simulink model "merohid"  (Simulink 7.6)
settings: Solver=ode45  StartTime=0.0  StopTime=10.0  RelTol=1e-3
libraries: fl_lib x6, elec_lib x1, nesl_utility x1
settings Model: Creator=Fodi  LastModifiedBy=Fodi

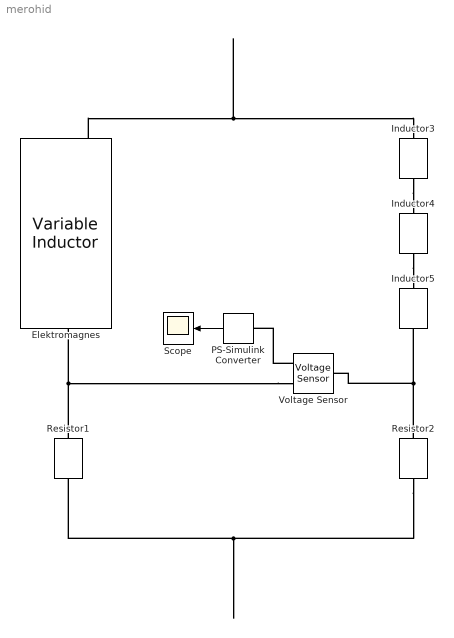
== system merohid ==
  Elektromagnes : elec_lib/Passive Devices/Variable Inductor  DialogController=NetworkEngine.DynNeDlgSource  SystemSampleTime=-1  prm=1  Lmin=1e-6 H  g=1e-9 1/Ohm  i0=0 A  phi0=0 Wb  LocalVarLogging=[]
  Inductor3 : fl_lib/Electrical/Electrical Elements/Inductor  DialogController=NetworkEngine.DynNeDlgSource  SystemSampleTime=-1  l=1e-6 H  i0=0 A  r=0 Ohm  g=1e-9 1/Ohm  i_Log=off  v_Log=off  i_L_Log=off  LocalVarNames=|i|v|i_L  LocalVarDescs=|i|v|Internal variable for current through inductor term  LocalVarLogging=[0 0 0]
  Inductor4 : fl_lib/Electrical/Electrical Elements/Inductor  DialogController=NetworkEngine.DynNeDlgSource  SystemSampleTime=-1  l=1e-6 H  i0=0 A  r=0 Ohm  g=1e-9 1/Ohm  i_Log=off  v_Log=off  i_L_Log=off  LocalVarNames=|i|v|i_L  LocalVarDescs=|i|v|Internal variable for current through inductor term  LocalVarLogging=[0 0 0]
  Inductor5 : fl_lib/Electrical/Electrical Elements/Inductor  DialogController=NetworkEngine.DynNeDlgSource  SystemSampleTime=-1  l=1e-6 H  i0=0 A  r=0 Ohm  g=1e-9 1/Ohm  i_Log=off  v_Log=off  i_L_Log=off  LocalVarNames=|i|v|i_L  LocalVarDescs=|i|v|Internal variable for current through inductor term  LocalVarLogging=[0 0 0]
  PS-Simulink Converter : nesl_utility/PS-Simulink Converter  DialogController=NetworkEngine.DynNeUtilDlgSource  SystemSampleTime=-1  PhysicalDomain=network_engine_domain  LeftPortType=input  RightPortType=output  SubClassName=ps_output  Unit=1  AffineConversion=off
  Resistor1 : fl_lib/Electrical/Electrical Elements/Resistor  DialogController=NetworkEngine.DynNeDlgSource  SystemSampleTime=-1  R=1 Ohm  i_Log=off  v_Log=off  LocalVarNames=|i|v  LocalVarDescs=|i|v  LocalVarLogging=[0 0]
  Resistor2 : fl_lib/Electrical/Electrical Elements/Resistor  DialogController=NetworkEngine.DynNeDlgSource  SystemSampleTime=-1  R=1 Ohm  i_Log=off  v_Log=off  LocalVarNames=|i|v  LocalVarDescs=|i|v  LocalVarLogging=[0 0]
  Scope : Scope
  Voltage Sensor : fl_lib/Electrical/Electrical Sensors/Voltage Sensor  DialogController=NetworkEngine.DynNeDlgSource  SystemSampleTime=-1  i1_Log=off  v1_Log=off  LocalVarNames=|i1|v1  LocalVarDescs=|i1|v1  LocalVarLogging=[0 0]
  wires:
  PS-Simulink Converter/1 -> Scope/1
  connections:
  Voltage Sensor/LConn1 -- Resistor2/LConn1 -- Inductor5/RConn1
  Elektromagnes/LConn2 -- Inductor3/LConn1
  Inductor3/RConn1 -- Inductor4/LConn1
  Inductor4/RConn1 -- Inductor5/LConn1
  Resistor2/RConn1 -- Resistor1/RConn1
  Voltage Sensor/RConn2 -- Resistor1/LConn1 -- Elektromagnes/RConn1
  Voltage Sensor/RConn1 -- PS-Simulink Converter/LConn1
